simulink model "FuelCellWorkBench"  (Simulink 7.9)
settings: Solver=ode1  StartTime=0.0  StopTime=max(pwr_profile(:,1))  FixedStep=1  RelTol=1e-3
undefined symbols (not defined in the file or in its folder): cyc_elevation_init
libraries: lib_fuel_cell x1
settings Model: Creator=mokeefe  LastModifiedBy=mokeefe
settings OptimizationCC: BooleanDataType=off
settings DebuggingCC: SaveWithParameterizedLinksMsg=none  SignalResolutionControl=TryResolveAllWithWarning  SolverPrmCheckMsg=none  MultiTaskDSMMsg=warning  MultiTaskCondExecSysMsg=none  StrictBusMsg=None
settings HardwareCC: TargetUnknown=on
settings RTWCC: IncludeERTFirstTime=on
settings GRTTargetCC: CombineOutputUpdateFcns=off  GRTInterface=on

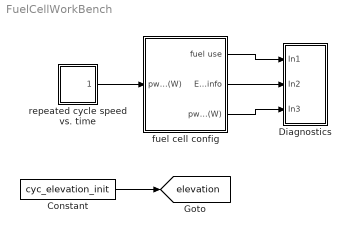
== system FuelCellWorkBench ==
  Constant : Constant  Value=cyc_elevation_init
  Diagnostics : Subsystem
  fuel cell config : Subsystem  BlockChoice=fuel converter <fc> VT model
      settings: AttributesFormatString=%<BlockChoice>  TemplateBlock=lib_fuel_cell/fuel cell config  MemberBlocks="fuel converter <fc>  KTH fc model,fuel converter <fc> GCTool linkage,fuel converter <fc> VT model,fuel converter <fc> net model,fuel converter <fc> polarization curve model"
  repeated cycle speed vs. time : Subsystem  mask(Repeating table){@1=pwr_profile(:,1), @2=pwr_profile(:,2)}
      mask prompts: @1 "Time values:"; @2 "Output values:"
      mask help:
      | Repeating table.
      | Enter values of time and output for first cycle.
      mask init:
      | period = max(@1); t = @1; y = @2;
      mask Help: Repeats cycle given in table. Time values should be monotonically increasing.
  tag scope: elevation=global
  wires:
  repeated cycle speed vs. time/1(out_1) -> fuel cell config/1(pwr req'd at fc  output (W))
  fuel cell config/1(fuel use) -> Diagnostics/1(In1)
  fuel cell config/2(EO emis info) -> Diagnostics/2(In2)
  fuel cell config/3(pwr avail. to driveline (W)) -> Diagnostics/3(In3)
  Constant/1 -> [elevation]

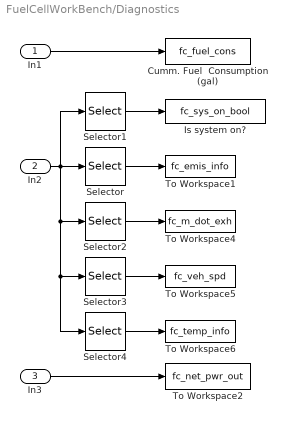
== system FuelCellWorkBench/Diagnostics ==
  In1 : Inport
  In2 : Inport  Port=2
  In3 : Inport  Port=3
  Cumm. Fuel  Consumption (gal) : ToWorkspace  VariableName=fc_fuel_cons  SampleTime=-1
  Is system on? : ToWorkspace  VariableName=fc_sys_on_bool  SampleTime=-1
  Selector : Selector  InputPortWidth=13  IndexOptions=Index vector (dialog)  Indices=[2 3 4 5 8]  OutputSizes=1
  Selector1 : Selector  InputPortWidth=13  IndexOptions=Index vector (dialog)  Indices=[1]  OutputSizes=1
  Selector2 : Selector  InputPortWidth=13  IndexOptions=Index vector (dialog)  Indices=[6]  OutputSizes=1
  Selector3 : Selector  InputPortWidth=13  IndexOptions=Index vector (dialog)  Indices=[8]  OutputSizes=1
  Selector4 : Selector  InputPortWidth=13  IndexOptions=Index vector (dialog)  Indices=[10 11 12 13 7]  OutputSizes=1
  To Workspace1 : ToWorkspace  VariableName=fc_emis_info  SampleTime=-1
  To Workspace2 : ToWorkspace  VariableName=fc_net_pwr_out  SampleTime=-1
  To Workspace4 : ToWorkspace  VariableName=fc_m_dot_exh  SampleTime=-1
  To Workspace5 : ToWorkspace  VariableName=fc_veh_spd  SampleTime=-1
  To Workspace6 : ToWorkspace  VariableName=fc_temp_info  SampleTime=-1
  wires:
  Selector4/1 -> To Workspace6/1
  Selector3/1 -> To Workspace5/1
  Selector2/1 -> To Workspace4/1
  Selector1/1 -> Is system on?/1
  Selector/1 -> To Workspace1/1
  In2/1 -> Selector4/1, Selector3/1, Selector2/1, Selector1/1, Selector/1
  In3/1 -> To Workspace2/1
  In1/1 -> Cumm. Fuel  Consumption (gal)/1

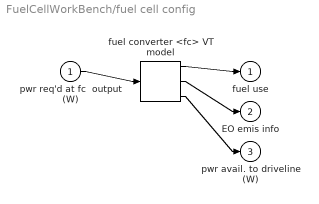
== system FuelCellWorkBench/fuel cell config ==
  pwr req'd at fc  output (W) : Inport
  fuel converter <fc> VT model : lib_fuel_cell/fuel converter <fc> VT model  SystemSampleTime=-1
  fuel use : Outport
  EO emis info : Outport  Port=2
  pwr avail. to driveline (W) : Outport  Port=3
  wires:
  pwr req'd at fc  output (W)/1 -> fuel converter <fc> VT model/1
  fuel converter <fc> VT model/1 -> fuel use/1
  fuel converter <fc> VT model/2 -> EO emis info/1
  fuel converter <fc> VT model/3 -> pwr avail. to driveline (W)/1

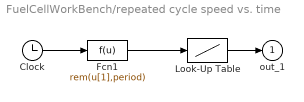
== system FuelCellWorkBench/repeated cycle speed vs. time ==
  Clock : Clock
  Fcn1 : Fcn  Expr=rem(u[1],period)
  Look-Up Table : Lookup  InputValues=t  Table=y  SaturateOnIntegerOverflow=on
  out_1 : Outport  InitialOutput=0
  wires:
  Fcn1/1 -> Look-Up Table/1
  Clock/1 -> Fcn1/1
  Look-Up Table/1 -> out_1/1
